simulink model "TwoNxInterleavedBoostConverter_AddedCapacitors"  (R2018a)
settings: Solver=ode23tb  StartTime=0.0  StopTime=0.1  MaxStep=1e-6  RelTol=1e-3
values from neighbouring files (symbols this model uses):
  C = 2.2e-6    (= 2.2e-06)    [parameter_set.m]
  L = 150e-6    (= 0.00015)    [parameter_set.m]
  WidthP = 60    [parameter_set.m]
libraries: powerlib x16, simulink x1
settings Model: Creator=Ilian  LastModifiedBy=ivank
settings SolverCC: InitialStep=1e-8  ZeroCrossAlgorithm=Adaptive
settings DebuggingCC: MaxConsecutiveZCsMsg=none  MaskedZcDiagnostic=none  IgnoredZcDiagnostic=none  UnconnectedInputMsg=none  UnconnectedOutputMsg=none  UnconnectedLineMsg=none

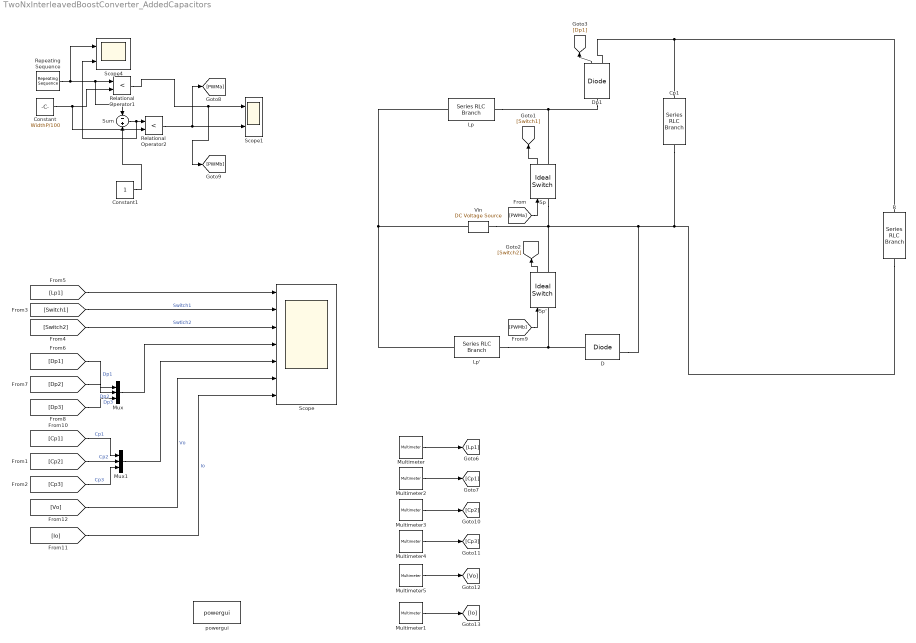
== system TwoNxInterleavedBoostConverter_AddedCapacitors ==
  "\tLp" : powerlib/Elements/Series RLC Branch  LConnTagsString=__new0  RConnTagsString=__new0  BranchType=L  Resistance=1  Inductance=L  SetiL0=off  InitialCurrent=0  Capacitance=1e-6  Setx0=off  InitialVoltage=0  Measurements=Branch voltage and current
  "\tR" : powerlib/Elements/Series RLC Branch  LConnTagsString=__new0  RConnTagsString=__new0  BranchType=R  Resistance=225  Inductance=150e-6  SetiL0=off  InitialCurrent=0  Capacitance=1e-6  Setx0=off  InitialVoltage=0  Measurements=Branch voltage and current
  Constant : Constant  Value=WidthP/100
  Constant1 : Constant
  Cp1 : powerlib/Elements/Series RLC Branch  LConnTagsString=__new0  RConnTagsString=__new0  BranchType=C  Resistance=1  Inductance=150e-3  SetiL0=off  InitialCurrent=0  Capacitance=C  Setx0=off  InitialVoltage=0  Measurements=Branch voltage and current
  D : powerlib/Power Electronics/Diode  Ron=0.001  Lon=0  Vf=VoltageDrop  IC=0  UseSnubber=0  Rs=500  Cs=250e-9  Measurements=on
  Dp1 : powerlib/Power Electronics/Diode  Ron=0.001  Lon=0  Vf=VoltageDrop  IC=0  UseSnubber=0  Rs=500  Cs=250e-9  Measurements=on
  Lp' : powerlib/Elements/Series RLC Branch  LConnTagsString=__new0  RConnTagsString=__new0  BranchType=L  Resistance=1  Inductance=L  SetiL0=off  InitialCurrent=0  Capacitance=1e-6  Setx0=off  InitialVoltage=0  Measurements=Branch voltage and current
  Multimeter : powerlib/Measurements/Multimeter  PhasorSimulation=off  OutputType=Complex  sel=1  L=8  Gain=1  yselected="{'Ub: \tLp'};"  PSBOutputType=1  PSBequivalent=0  AxesSetting=[0,0.1,-100,100]  Display=0  SavedBlockNames=-11
  Multimeter1 : powerlib/Measurements/Multimeter  PhasorSimulation=off  OutputType=Complex  sel=6  L=8  Gain=1  yselected="{'Ib: \tR'};"  PSBOutputType=1  PSBequivalent=0  AxesSetting=[0,0.1,-100,100]  Display=0  SavedBlockNames=-11
  Multimeter2 : powerlib/Measurements/Multimeter  PhasorSimulation=off  OutputType=Complex  sel=3  L=8  Gain=1  yselected={'Ub: Cp1'};  PSBOutputType=1  PSBequivalent=0  AxesSetting=[0,0.1,-100,100]  Display=0  SavedBlockNames=-11
  Multimeter3 : powerlib/Measurements/Multimeter  PhasorSimulation=off  OutputType=Complex  sel=1  L=8  Gain=0  yselected={}  PSBOutputType=1  PSBequivalent=0  AxesSetting=[0,0.1,-100,100]  Display=0  SavedBlockNames=-11
  Multimeter4 : powerlib/Measurements/Multimeter  PhasorSimulation=off  OutputType=Complex  sel=1  L=8  Gain=0  yselected={}  PSBOutputType=1  PSBequivalent=0  AxesSetting=[0,0.1,-100,100]  Display=0  SavedBlockNames=-11
  Multimeter5 : powerlib/Measurements/Multimeter  PhasorSimulation=off  OutputType=Complex  sel=2  L=8  Gain=1  yselected="{'Ub: \tR'};"  PSBOutputType=1  PSBequivalent=0  AxesSetting=[0,0.1,-100,100]  Display=0  SavedBlockNames=-11
  Mux : Mux  Inputs=3
  Mux1 : Mux  Inputs=3
  Relational Operator1 : RelationalOperator  Operator=<  OutDataTypeStr=boolean  RndMeth=Simplest
  Relational Operator2 : RelationalOperator  Operator=<  OutDataTypeStr=boolean  RndMeth=Simplest
  Repeating Sequence : simulink/Sources/Repeating Sequence  rep_seq_t=[0 1/2 1]*(1/50000)  rep_seq_y=[0 1 0]
  Scope : Scope  NumInputPorts=7
  Scope1 : Scope  NumInputPorts=2
  Scope4 : Scope  NumInputPorts=2
  Sp : powerlib/Power Electronics/Ideal Switch  Ron=R_internal  Lon=0  IC=0  Rs=1e5  Cs=inf  Measurements=on
  Sp' : powerlib/Power Electronics/Ideal Switch  Ron=R_internal  Lon=0  IC=0  Rs=1e5  Cs=inf  Measurements=on
  Sum : Sum  Inputs=-+
  Vin : powerlib/Electrical Sources/DC Voltage Source  Amplitude=10  Measurements=None
  powergui : powerlib/powergui  Priority=1  SimulationMode=Continuous  SampleTime=50e-6  frequency=60  Iterations=50  frequencyindice=0  Pbase=100e6  ErrMax=1e-4  UnitsV=kV  UnitsW=MW  buscounter=0  FunctionMessages=off  echomessages=off  EnableUseOfTLC=off  CurrentSourceSwitches=off  DisableSnubberDevices=off  DisableRonSwitches=off  DisableVfSwitches=off  DisplayEquations=off  SolverType=Tustin/Backward Euler (TBE)  Interpol=off  ExternalGateDelay=off  methode=off  Ts=100  x0status=blocks  SPID=on  SwTol=0  HookPort=off  RestoreLinks=warning  ResistiveCurrentMeasurement=off  Frange=[0:2:500]  Ylog=off  Xlog=on  ShowGrid=off  save=off  variable=ZData  structure=0  ZoomFFT=off  StartTime=0.0  cycles=1  DisplayStyle=1  fundamental=60  FreqAxis=off  MaxFrequency=1000  frequencyindicesteady=1  RmsSteady=1  display=off
  wires:
  Relational Operator2/1 -> [PWMa], Scope1/2
  Constant1/1 -> Sum/2
  Sum/1 -> Scope4/2, Relational Operator2/1
  Constant/1 -> Relational Operator2/2, Relational Operator1/2
  Repeating Sequence/1 -> Scope4/1, Sum/1, Relational Operator1/1
  Relational Operator1/1 -> [PWMb], Scope1/1
  [PWMa] -> Sp/1
  [PWMb] -> Sp'/1
  Sp/1 -> [Switch1]
  Sp'/1 -> [Switch2]
  [Switch1] -> Scope/2  "Switch1"
  [Lp1] -> Scope/1
  Dp1/1 -> [Dp1]
  Multimeter/1 -> [Lp1]
  Multimeter2/1 -> [Cp1]
  Multimeter4/1 -> [Cp3]
  Multimeter3/1 -> [Cp2]
  [Switch2] -> Scope/3  "Swtich2"
  [Dp1] -> Mux/1  "Dp1"
  [Dp2] -> Mux/2  "Dp2"
  [Dp3] -> Mux/3  "Dp3"
  Mux/1 -> Scope/4
  [Cp1] -> Mux1/1  "Cp1"
  [Cp2] -> Mux1/2  "Cp2"
  [Cp3] -> Mux1/3  "Cp3"
  Mux1/1 -> Scope/5
  Multimeter5/1 -> [Vo]
  [Vo] -> Scope/6  "Vo"
  Multimeter1/1 -> [Io]
  [Io] -> Scope/7  "Io"
  connections:
  Vin/RConn1 -- Lp'/LConn1 -- "\tLp"/LConn1
  "\tLp"/RConn1 -- Dp1/LConn1 -- Sp/RConn1
  Dp1/RConn1 -- "\tR"/LConn1 -- Cp1/LConn1
  Cp1/RConn1 -- Sp/LConn1 -- Sp'/RConn1 -- Vin/LConn1 -- D/RConn1 -- "\tR"/RConn1
  Lp'/RConn1 -- Sp'/LConn1 -- D/LConn1
